simulink library "ACC_L2"  (R2024b)
settings: Solver=VariableStepAuto  StartTime=0.0  StopTime=10.0  RelTol=1e-3

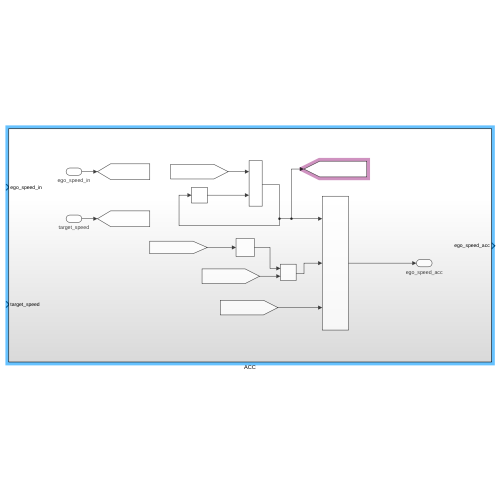
[thumbnail: Simulink's stored preview of the top-level diagram]
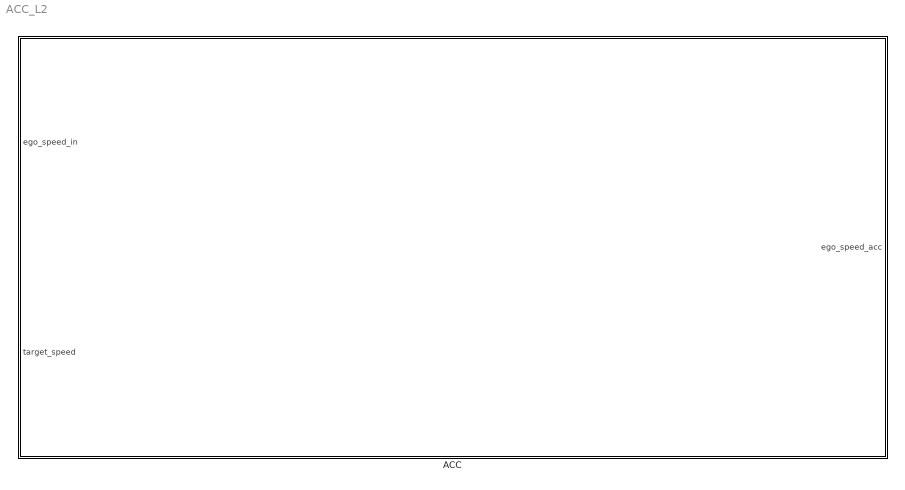
== system ACC_L2 ==
  ACC : Subsystem

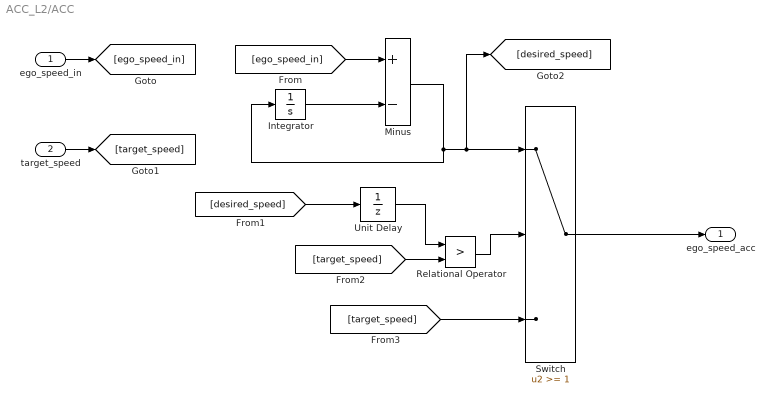
== system ACC_L2/ACC ==
  ego_speed_in : Inport
  target_speed : Inport  Port=2
  Integrator : Integrator
  Minus : Sum  Inputs=+-
  Relational Operator : RelationalOperator  Operator=>  OutDataTypeStr=boolean  RndMeth=Simplest  InputSameDT=off
  Switch : Switch  Threshold=1  SaturateOnIntegerOverflow=off  InputSameDT=off
  Unit Delay : UnitDelay  SampleTime=-1  HasFrameUpgradeWarning=on
  ego_speed_acc : Outport
  wires:
  Switch/1 -> ego_speed_acc/1
  Unit Delay/1 -> Relational Operator/1
  Relational Operator/1 -> Switch/2
  Integrator/1 -> Minus/2
  [target_speed] -> Relational Operator/2
  [target_speed] -> Switch/3
  [ego_speed_in] -> Minus/1
  [desired_speed] -> Unit Delay/1
  target_speed/1 -> [target_speed]
  ego_speed_in/1 -> [ego_speed_in]
  Minus/1 -> Integrator/1, Switch/1, [desired_speed]
